simulink model "DrivetrainHevIps"  (R2018a)
settings: Solver=VariableStepAuto  StartTime=0.0  StopTime=inf  RelTol=1e-3  EnableMultiTasking=on
model workspace (MAT data in the model file):
  DiffRatio = 3.267
  Jc1 = 0.2
  Jp1 = 0.01
  Jr1 = 0.03
  Js1 = 0.01
  NF = Simulink.Parameter
  NF.Value = 2
  NF.DataType = 'auto'
  NF.Dimensions = [1 1]
  NR = Simulink.Parameter
  NR.Value = 2
  NR.DataType = 'auto'
  NR.Dimensions = [1 1]
  Np1 = 23
  Np2 = 18
  Nr1 = 78
  Nr2 = 58
  Ns1 = 30
  Ns2 = 22
  RWheel = 0.31075
  b_axle = Simulink.Parameter
  b_axle.Value = 10
  b_axle.DataType = 'auto'
  b_axle.Dimensions = [1 1]
  b_driveshaft = Simulink.Parameter
  b_driveshaft.Value = 10
  b_driveshaft.DataType = 'auto'
  b_driveshaft.Dimensions = [1 1]
  bc1 = 0.005
  bp1 = 0.005
  br1 = 0.005
  bs1 = 0.005
  k_axle = Simulink.Parameter
  k_axle.Value = 5000
  k_axle.DataType = 'auto'
  k_axle.Dimensions = [1 1]
  k_driveshaft = Simulink.Parameter
  k_driveshaft.Value = 1000
  k_driveshaft.DataType = 'auto'
  k_driveshaft.Dimensions = [1 1]
  wc_shaft = Simulink.Parameter
  wc_shaft.Value = 50
  wc_shaft.DataType = 'auto'
  wc_shaft.Dimensions = [1 1]
libraries: autolibsharedcoupling x7, autolibshared x7, autolibshareddiff x4, autolibcoupling x2
(part 1 of 4)
settings Model: ModifiedByFormat=The MathWorks, Inc.  SimulationMode=accelerator  PauseTimes=10  Creator=The MathWorks, Inc.  LastModifiedBy=The MathWorks, Inc.
settings SolverCC: DecoupledContinuousIntegration=on
settings DataIOCC: DSMLogging=off
settings ModelReferenceCC: PropagateSignalLabelsOutOfModel=off
settings CodeAppCC: StateflowObjectComments=on
settings GRTTargetCC: TargetLangStandard=C89/C90 (ANSI)
settings ConfigComp: CovMetricSettings=dsw  CovHtmlReporting=on  CovSaveCumulativeToWorkspaceVar=on  CovSaveSingleToWorkspaceVar=on  CovShowResultsExplorer=off  CovExternalEMLEnable=off
settings SimscapeCC: SimscapeNormalizeSystem=off  SimscapeNominalValues={1, 'bar'; 1, 'cm^3/s'; 1, 'bar*kg/s'; 1, 'kJ/kg'; 1, 'kW'; }

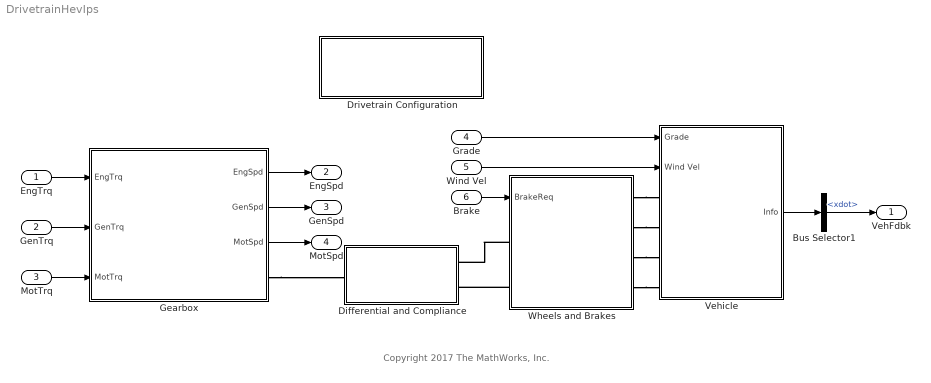
== system DrivetrainHevIps ==
  note: Copyright 2017 The MathWorks, Inc.
  EngTrq : Inport
  GenTrq : Inport  Port=2
  MotTrq : Inport  Port=3
  Grade : Inport  Port=4
  Wind Vel : Inport  Port=5
  Brake : Inport  Port=6
  Bus Selector1 : BusSelector  OutputSignals=BdyFrm.Cg.Vel.xdot
  Differential and Compliance : Subsystem  Variant=on  OverrideUsingVariant=0
  Drivetrain Configuration : Subsystem  mask(Drivetrain Configuration){drivetrainMode=Front Wheel Drive}
      mask prompts: drivetrainMode "Drivetrain Mode"
      mask help: Use this block to configure the dirvetrain mode.
      settings: AttributesFormatString=Active Mode: %<drivetrainMode>
      mask TypeOptions drivetrainMode: Front Wheel Drive | Rear Wheel Drive | All Wheel Drive
      mask Callback drivetrainMode:
      | switch get_param(gcb,'drivetrainMode')
      |     case 'Front Wheel Drive'
      |         set_param([bdroot '/Wheels and Brakes'],'OverrideUsingVariant','0')
      |         set_param([bdroot '/Differential and Compliance'],'OverrideUsingVariant','0')
      |     case 'Rear Wheel Drive'
      |         set_param([bdroot '/Wheels and Brakes'],'OverrideUsingVariant','1')
      |         set_param([bdroot '/Differential and Compliance'],'OverrideUsingVariant','1')
      |     case 'All Wheel Drive'
      |         set_param([bdroot '/Wheels and Brakes'],'OverrideUsingVariant','2')
      |         set_param([bdroot '/Differential and Compliance'],'OverrideUsingVariant','2')
      |     otherwise
      |         set_param([bdroot '/Wheels and Brakes'],'OverrideUsingVariant','0')
      |         set_param([bdroot '/Differential and Compliance'],'OverrideUsingVariant','0')
      | end
      mask Display: disp('Double click to configure drivetrain')
  Gearbox : Subsystem
  Vehicle : Subsystem
  Wheels and Brakes : Subsystem  Variant=on  OverrideUsingVariant=0
  VehFdbk : Outport
  EngSpd : Outport  Port=2  BusOutputAsStruct=on
  GenSpd : Outport  Port=3  BusOutputAsStruct=on
  MotSpd : Outport  Port=4  BusOutputAsStruct=on
  wires:
  Brake/1 -> Wheels and Brakes/1(BrakeReq)
  EngTrq/1 -> Gearbox/1(EngTrq)
  GenTrq/1 -> Gearbox/2(GenTrq)
  MotTrq/1 -> Gearbox/3(MotTrq)
  Vehicle/1(Info) -> Bus Selector1/1
  Bus Selector1/1 -> VehFdbk/1  "<xdot>"
  Grade/1 -> Vehicle/1(Grade)
  Wind Vel/1 -> Vehicle/2(Wind Vel)
  Gearbox/1(EngSpd) -> EngSpd/1
  Gearbox/2(GenSpd) -> GenSpd/1
  Gearbox/3(MotSpd) -> MotSpd/1
  connections:
  Wheels and Brakes/RConn2 -- Vehicle/LConn2
  Wheels and Brakes/RConn1 -- Vehicle/LConn1
  Wheels and Brakes/RConn4 -- Vehicle/LConn4
  Wheels and Brakes/RConn3 -- Vehicle/LConn3
  Gearbox/RConn1 -- Differential and Compliance/LConn1
  Wheels and Brakes/LConn1 -- Differential and Compliance/RConn1
  Wheels and Brakes/LConn2 -- Differential and Compliance/RConn2

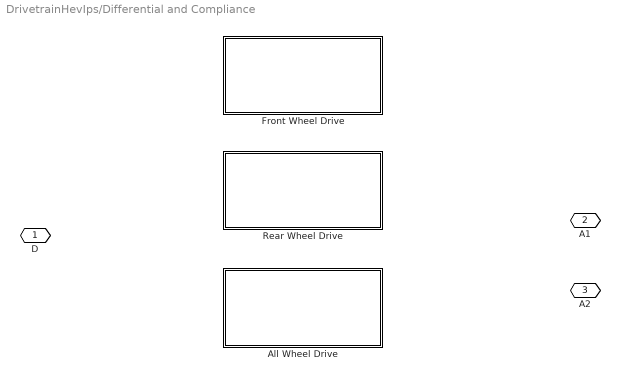
== system DrivetrainHevIps/Differential and Compliance ==
  All Wheel Drive : Subsystem  VariantControl=2
  Front Wheel Drive : Subsystem  VariantControl=0
  Rear Wheel Drive : Subsystem  VariantControl=1
  D : PMIOPort  Side=Left
  A1 : PMIOPort  Port=2  Side=Right
  A2 : PMIOPort  Port=3  Side=Right

== system DrivetrainHevIps/Drivetrain Configuration ==

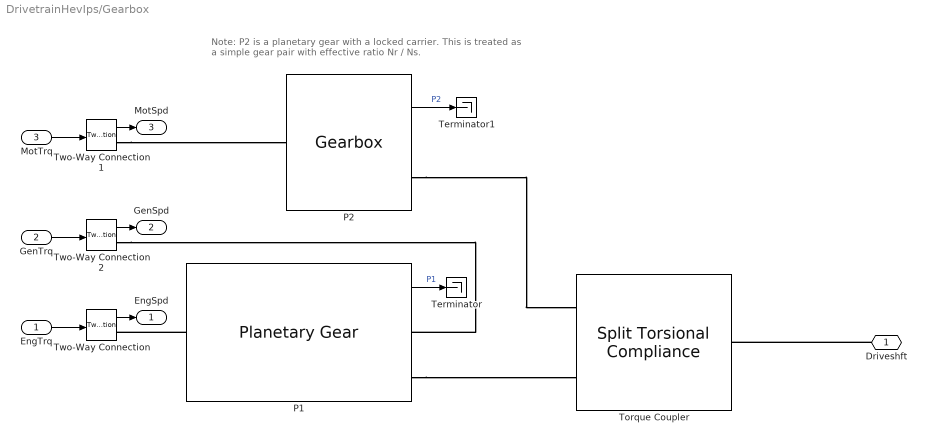
== system DrivetrainHevIps/Gearbox ==
  note: Note: P2 is a planetary gear with a locked carrier.
      | This is treated as a simple gear pair with effective ratio Nr / Ns.
  EngTrq : Inport
  GenTrq : Inport  Port=2
  MotTrq : Inport  Port=3
  P1 : autolibcoupling/Planetary Gear  port_config=Two-way connection  input_config=Torque input - velocity output  Nsp=Ns1/Np1  Nsr=Ns1/Nr1  Js=Js1  Jp=Jp1  Jr=Jr1  Jc=Jc1  bs=bs1  br=br1  bp=bp1  bc=bc1  ws_o=0  wc_o=0  blkID=0
      settings: SourceProductName=Powertrain Blockset  SourceProductBaseCode=PW
  P2 : autolibcoupling/Gearbox  port_config=Two-way connection  input_config=Torque input - velocity output  dirSwitch=on  N=Nr2/Ns2  J1=.01  J2=.01  b1=0.005  b2=0.005  theta1_o=0  w1_o=0  blkID=0
      settings: SourceProductName=Powertrain Blockset  SourceProductBaseCode=PW
  Terminator : Terminator
  Terminator1 : Terminator
  Torque Coupler : autolibsharedcoupling/Split Torsional Compliance  port_config=Two-way connection  cplrMode=Shaft merge  k1=k_axle  b1=b_axle  omega1_c=50  theta1_o=0  domega1_o=0  k2=k_axle  b2=b_axle  omega2_c=50  theta2_o=0  domega2_o=0  blkID=0  aMode=1
      settings: SourceProductName=Powertrain Blockset  SourceProductBaseCode=PW
  Two-Way Connection : TwoWayConnection
  Two-Way Connection1 : TwoWayConnection
  Two-Way Connection2 : TwoWayConnection
  Driveshft : PMIOPort  Side=Right
  EngSpd : Outport
  GenSpd : Outport  Port=2
  MotSpd : Outport  Port=3
  wires:
  P2/1 -> Terminator1/1  "P2"
  EngTrq/1 -> Two-Way Connection/1
  Two-Way Connection/1 -> EngSpd/1
  GenTrq/1 -> Two-Way Connection2/1
  P1/1 -> Terminator/1  "P1"
  Two-Way Connection1/1 -> MotSpd/1
  MotTrq/1 -> Two-Way Connection1/1
  Two-Way Connection2/1 -> GenSpd/1
  connections:
  P1/RConn2 -- Torque Coupler/LConn2
  P1/LConn1 -- Two-Way Connection/RConn1
  Two-Way Connection2/RConn1 -- P1/RConn1
  Two-Way Connection1/RConn1 -- P2/LConn1
  P2/RConn1 -- Torque Coupler/LConn1
  Driveshft/RConn1 -- Torque Coupler/RConn1

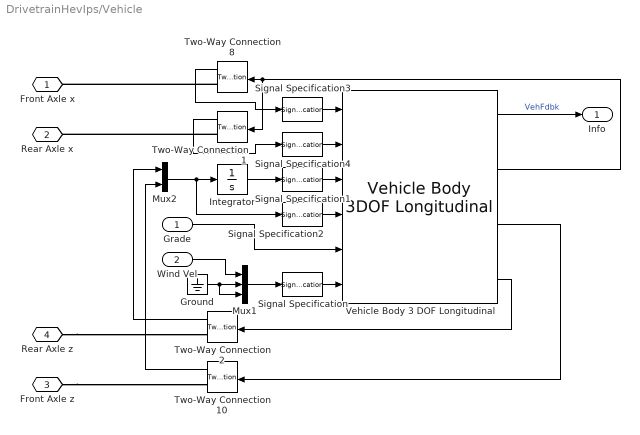
== system DrivetrainHevIps/Vehicle ==
  Grade : Inport  Unit=deg
  Wind Vel : Inport  Port=2  Unit=m/s
  Ground : Ground
  Integrator : Integrator
  Mux1 : Mux  Inputs=3
  Mux2 : Mux  Inputs=2
  Signal Specification : SignalSpecification  Unit=m/s
  Signal Specification1 : SignalSpecification  Unit=m
  Signal Specification2 : SignalSpecification  Unit=m/s
  Signal Specification3 : SignalSpecification  Unit=N
  Signal Specification4 : SignalSpecification  Unit=N
  Two-Way Connection{1..2,8,10} (4 alike) : TwoWayConnection
  Vehicle Body 3 DOF Longitudinal : autolibshared/Vehicle Body 3DOF Longitudinal  VariantControl=SL  groundType=Axle displacement, velocity  aMode=1  NF=NF  NR=NR  m=1310  a=1.08  b=1.62  h=.5  Cd=0.25  Af=2.27  x_o=0  xdot_o=0  Cl=.1  z_o=-0.298  zdot_o=0  Iyy=3000  Cpm=.1  theta_o=0  q_o=0  FskF=[-50, -1, 0, 2, 3, 52].*1.25e4 / 70  dzsF=[-5e-3, -1e-4, 0, .2, .2001, .2051]  FsbF=[-10000 -100 -10 0 10 100 10000] * 70  dzdotsF=[-10 -1 -.1 0 .1 1 10]  FskR=[-50, -1, 0, 2, 3, 52].*7.5e3 / 70  dzsR=[-5e-3, -1e-4, 0, .2, .2001, .2051]  FsbR=[-10000 -100 -10 0 10 100 10000] * 70  dzdotsR=[-10 -1 -.1 0 .1 1 10]  Pabs=101325  T=273  g=9.81  blkID=0
      settings: SourceProductName=Powertrain Blockset  SourceProductBaseCode=PW
  Front Axle x : PMIOPort  Side=Left
  Rear Axle x : PMIOPort  Port=2  Side=Left
  Front Axle z : PMIOPort  Port=3  Side=Left
  Rear Axle z : PMIOPort  Port=4  Side=Left
  Info : Outport
  wires:
  Vehicle Body 3 DOF Longitudinal/3 -> Two-Way Connection10/1
  Two-Way Connection8/1 -> Signal Specification3/1
  Vehicle Body 3 DOF Longitudinal/1 -> Info/1  "VehFdbk"
  Ground/1 -> Mux1/2, Mux1/3
  Mux1/1 -> Signal Specification/1
  Two-Way Connection1/1 -> Signal Specification4/1
  Vehicle Body 3 DOF Longitudinal/4 -> Two-Way Connection2/1
  Two-Way Connection2/1 -> Mux2/1
  Two-Way Connection10/1 -> Mux2/2
  Mux2/1 -> Signal Specification2/1, Integrator/1
  Integrator/1 -> Signal Specification1/1
  Wind Vel/1 -> Mux1/1
  Signal Specification1/1 -> Vehicle Body 3 DOF Longitudinal/3
  Signal Specification4/1 -> Vehicle Body 3 DOF Longitudinal/2
  Signal Specification3/1 -> Vehicle Body 3 DOF Longitudinal/1
  Vehicle Body 3 DOF Longitudinal/2 -> Two-Way Connection1/1, Two-Way Connection8/1
  Signal Specification2/1 -> Vehicle Body 3 DOF Longitudinal/4
  Grade/1 -> Vehicle Body 3 DOF Longitudinal/5
  Signal Specification/1 -> Vehicle Body 3 DOF Longitudinal/6
  connections:
  Two-Way Connection8/RConn1 -- Front Axle x/RConn1
  Front Axle z/RConn1 -- Two-Way Connection10/RConn1
  Two-Way Connection1/RConn1 -- Rear Axle x/RConn1
  Rear Axle z/RConn1 -- Two-Way Connection2/RConn1

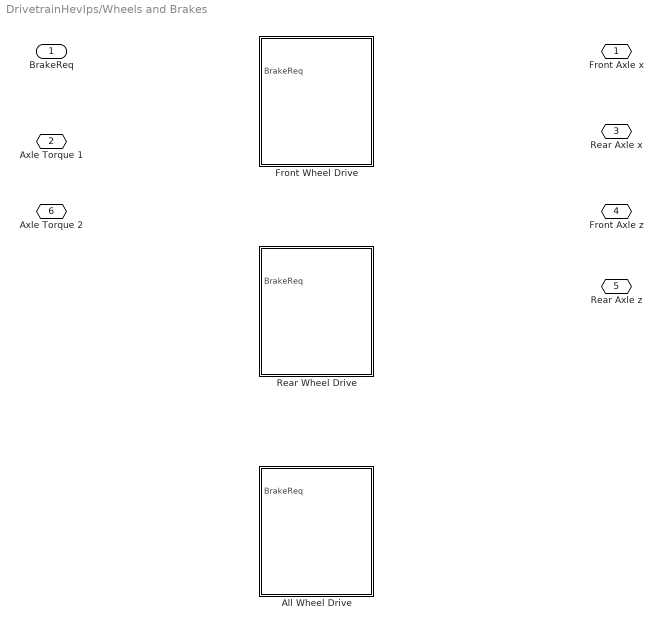
== system DrivetrainHevIps/Wheels and Brakes ==
  BrakeReq : Inport
  All Wheel Drive : Subsystem  VariantControl=2
  Front Wheel Drive : Subsystem  VariantControl=0
  Rear Wheel Drive : Subsystem  VariantControl=1
  Front Axle x : PMIOPort  Side=Right
  Axle Torque 1 : PMIOPort  Port=2  Side=Left
  Rear Axle x : PMIOPort  Port=3  Side=Right
  Front Axle z : PMIOPort  Port=4  Side=Right
  Rear Axle z : PMIOPort  Port=5  Side=Right
  Axle Torque 2 : PMIOPort  Port=6  Side=Left

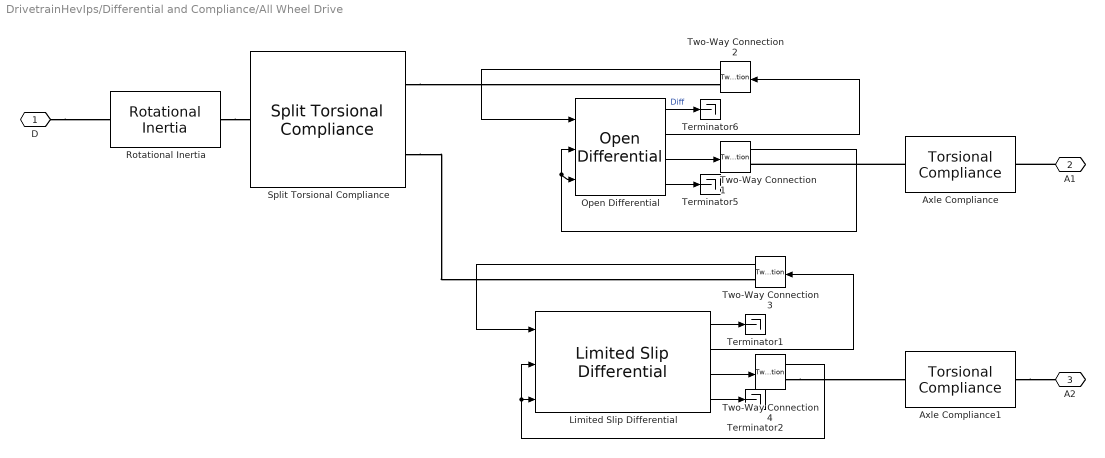
== system DrivetrainHevIps/Differential and Compliance/All Wheel Drive ==
  Axle Compliance : autolibsharedcoupling/Torsional Compliance  port_config=Two-way connection  k=k_axle  b=b_axle  theta_o=0  domega_o=0  omega_c=wc_shaft  blkID=0  aMode=1
      settings: SourceProductName=Powertrain Blockset
  Axle Compliance1 : autolibsharedcoupling/Torsional Compliance  port_config=Two-way connection  k=k_axle  b=b_axle  theta_o=0  domega_o=0  omega_c=wc_shaft  blkID=0  aMode=1
      settings: SourceProductName=Powertrain Blockset
  Limited Slip Differential : autolibshareddiff/Limited Slip Differential  shaftSwitchMask=To the left of center-line  Ndiff=DiffRatio  Jd=.025  bd=1e-3  Jw1=.01  bw1=1e-3  Jw2=.01  bw2=1e-3  omegaw1o=0  omegaw2o=0  couplingType=Pre-loaded ideal clutch  Ndisks=4  Reff=.20  Fc=500  muc=[.16 0.13 0.115 0.11 0.105 0.1025 0.10125]  dw=[0 10 20 40 60 80 100]  Tdw=[-100, -90, -50, -5, 0, 5, 50, 90, 100]  dwT=[-200, -175, -100, - 50, 0, 50, 100, 175, 200]  TTin=[-200 -175 -100 - 50 0 50 100 175 200]  Tin=[-200 -175 -100 - 50 0 50 100 175 200]  tauC=.01  IdealInterpMethod=Linear  IdealExtrapMethod=Linear  TdwInterpMethod=Linear  TdwExtrapMethod=Linear  TTinInterpMethod=Linear  TTinExtrapMethod=Linear  maxAbsSpd=5e3  aMode=1
      settings: SourceProductName=Powertrain Blockset  SourceProductBaseCode=PW
  Open Differential : autolibshareddiff/Open Differential  shaftSwitchMask=To the left of center-line  Ndiff=DiffRatio  Jd=.025  bd=1e-3  Jw1=.01  bw1=1e-3  Jw2=.01  bw2=1e-3  omegaw1o=0  omegaw2o=0  maxAbsSpd=5e3  aMode=1
      settings: SourceProductName=Powertrain Blockset
  Rotational Inertia : autolibsharedcoupling/Rotational Inertia  port_config=Two-way connection  J=.01  b=.001  omega_o=0  externJ=off  blkID=0  aMode=1
      settings: SourceProductName=Powertrain Blockset  SourceProductBaseCode=PW
  Split Torsional Compliance : autolibsharedcoupling/Split Torsional Compliance  port_config=Two-way connection  cplrMode=Shaft split  k1=5e4  b1=1e2  omega1_c=3000  theta1_o=0  domega1_o=0  k2=5e4  b2=1e2  omega2_c=3000  theta2_o=0  domega2_o=0  blkID=0  aMode=1
      settings: SourceProductName=Powertrain Blockset  SourceProductBaseCode=PW
  Terminator{1..2,5..6} (4 alike) : Terminator
  Two-Way Connection{1..4} (4 alike) : TwoWayConnection
  D : PMIOPort  Side=Left
  A1 : PMIOPort  Port=2  Side=Right
  A2 : PMIOPort  Port=3  Side=Right
  wires:
  Open Differential/1 -> Terminator6/1  "Diff"
  Two-Way Connection2/1 -> Open Differential/1
  Two-Way Connection1/1 -> Open Differential/3, Open Differential/2
  Open Differential/3 -> Two-Way Connection1/1
  Open Differential/4 -> Terminator5/1
  Open Differential/2 -> Two-Way Connection2/1
  Two-Way Connection3/1 -> Limited Slip Differential/1
  Limited Slip Differential/1 -> Terminator1/1
  Limited Slip Differential/3 -> Two-Way Connection4/1
  Two-Way Connection4/1 -> Limited Slip Differential/3, Limited Slip Differential/2
  Limited Slip Differential/2 -> Two-Way Connection3/1
  Limited Slip Differential/4 -> Terminator2/1
  connections:
  D/RConn1 -- Rotational Inertia/LConn1
  Split Torsional Compliance/RConn1 -- Two-Way Connection2/RConn1
  Axle Compliance/LConn1 -- Two-Way Connection1/RConn1
  A1/RConn1 -- Axle Compliance/RConn1
  Split Torsional Compliance/RConn2 -- Two-Way Connection3/RConn1
  Axle Compliance1/RConn1 -- A2/RConn1
  Two-Way Connection4/RConn1 -- Axle Compliance1/LConn1
  Rotational Inertia/RConn1 -- Split Torsional Compliance/LConn1

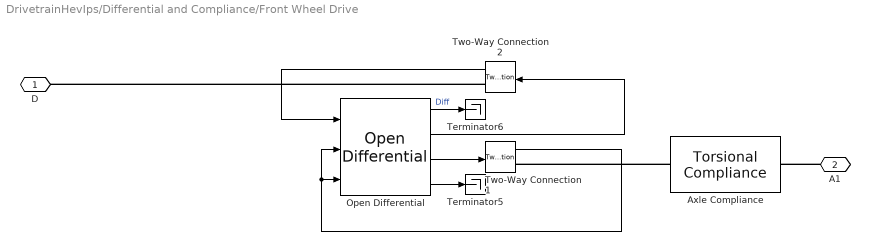
== system DrivetrainHevIps/Differential and Compliance/Front Wheel Drive ==
  Axle Compliance : autolibsharedcoupling/Torsional Compliance  port_config=Two-way connection  k=k_axle  b=b_axle  theta_o=0  domega_o=0  omega_c=wc_shaft  blkID=0  aMode=1
      settings: SourceProductName=Powertrain Blockset
  Open Differential : autolibshareddiff/Open Differential  shaftSwitchMask=To the left of center-line  Ndiff=DiffRatio  Jd=.025  bd=1e-3  Jw1=.01  bw1=1e-3  Jw2=.01  bw2=1e-3  omegaw1o=0  omegaw2o=0  maxAbsSpd=5e3  aMode=1
      settings: SourceProductName=Powertrain Blockset
  Terminator5 : Terminator
  Terminator6 : Terminator
  Two-Way Connection1 : TwoWayConnection
  Two-Way Connection2 : TwoWayConnection
  D : PMIOPort  Side=Left
  A1 : PMIOPort  Port=2  Side=Right
  wires:
  Open Differential/1 -> Terminator6/1  "Diff"
  Two-Way Connection2/1 -> Open Differential/1
  Two-Way Connection1/1 -> Open Differential/3, Open Differential/2
  Open Differential/3 -> Two-Way Connection1/1
  Open Differential/4 -> Terminator5/1
  Open Differential/2 -> Two-Way Connection2/1
  connections:
  A1/RConn1 -- Axle Compliance/RConn1
  Axle Compliance/LConn1 -- Two-Way Connection1/RConn1
  Two-Way Connection2/RConn1 -- D/RConn1

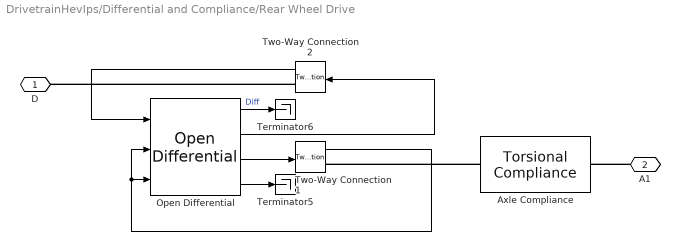
== system DrivetrainHevIps/Differential and Compliance/Rear Wheel Drive ==
  Axle Compliance : autolibsharedcoupling/Torsional Compliance  port_config=Two-way connection  k=k_axle  b=b_axle  theta_o=0  domega_o=0  omega_c=wc_shaft  blkID=0  aMode=1
      settings: SourceProductName=Powertrain Blockset
  Open Differential : autolibshareddiff/Open Differential  shaftSwitchMask=To the left of center-line  Ndiff=DiffRatio  Jd=.025  bd=1e-3  Jw1=.01  bw1=1e-3  Jw2=.01  bw2=1e-3  omegaw1o=0  omegaw2o=0  maxAbsSpd=5e3  aMode=1
      settings: SourceProductName=Powertrain Blockset
  Terminator5 : Terminator
  Terminator6 : Terminator
  Two-Way Connection1 : TwoWayConnection
  Two-Way Connection2 : TwoWayConnection
  D : PMIOPort  Side=Left
  A1 : PMIOPort  Port=2  Side=Right
  wires:
  Open Differential/1 -> Terminator6/1  "Diff"
  Two-Way Connection2/1 -> Open Differential/1
  Two-Way Connection1/1 -> Open Differential/3, Open Differential/2
  Open Differential/3 -> Two-Way Connection1/1
  Open Differential/4 -> Terminator5/1
  Open Differential/2 -> Two-Way Connection2/1
  connections:
  A1/RConn1 -- Axle Compliance/RConn1
  Axle Compliance/LConn1 -- Two-Way Connection1/RConn1
  Two-Way Connection2/RConn1 -- D/RConn1
